simulink model "bike_model_pidTuning"  (R2018b)
settings: Solver=FixedStepAuto  StartTime=0.0  StopTime=sim_time  FixedStep=Ts_IMU  MaxStep=Ts  RelTol=1e-3
values from neighbouring files (symbols this model uses):
  a_compFilter = a_real    (= 0.4964)    [configuration_boxMovedCenter.m]    (also in configuration_lqrTuning.m = 0.325; configuration_pidTuning.m = 0.325; configuration_yixiao.m = 0.325)
  b_compFilter = b_real    (= 1.095)    [configuration_boxMovedCenter.m]    (also in configuration_lqrTuning.m; configuration_pidTuning.m; configuration_yixiao.m)
  b_real = 1.095    [configuration_boxMovedCenter.m]    (also in configuration_lqrTuning.m; configuration_pidTuning.m; configuration_yixiao.m)
  direct_control = 1    [configuration_boxMovedCenter.m]    (also in configuration_lqrTuning.m; configuration_pidTuning.m; configuration_yixiao.m)
  IMU_height_real = 0.45    [configuration_boxMovedCenter.m]    (also in configuration_lqrTuning.m; configuration_pidTuning.m; configuration_yixiao.m)
  initial_states = [deg2rad(5) deg2rad(-2) deg2rad(0)]    [configuration_boxMovedCenter.m]    (also in configuration_lqrTuning.m = [deg2rad(-2) deg2rad(0) deg2rad(0)]; configuration_pidTuning.m = [deg2rad(-2) deg2rad(0) deg2rad(0)]; configuration_yixiao.m = [deg2rad(-2) deg2rad(0) deg2rad(0)])
  input_velocity = 3    [configuration_boxMovedCenter.m]    (also in configuration_lqrTuning.m; configuration_pidTuning.m; configuration_yixiao.m)
  lambda_compFilter = deg2rad(70)    [configuration_boxMovedCenter.m]    (also in configuration_lqrTuning.m; configuration_pidTuning.m; configuration_yixiao.m)
  lambda_real = deg2rad(70)    [configuration_boxMovedCenter.m]    (also in configuration_lqrTuning.m; configuration_pidTuning.m; configuration_yixiao.m)
  look_ahead = 0    [configuration_boxMovedCenter.m]    (also in configuration_lqrTuning.m; configuration_pidTuning.m; configuration_yixiao.m)
  parameters_compFilter = [g h_compFilter b_compFilter a_compFilter lambda_compFilter c_compFilter]    [configuration_boxMovedCenter.m]    (also in configuration_lqrTuning.m; configuration_pidTuning.m; configuration_yixiao.m)
  parameters_f_b_real = [m_frame_real m_box_real h_frame_real h_box_real a_frame_real a_box_real c_frame_real c_box_real b_frame_real b_box_real l_frame_real l_box_real]    [configuration_boxMovedCenter.m]    (also in configuration_lqrTuning.m; configuration_pidTuning.m; configuration_yixiao.m = [m_frame_real m_box_real h_frame_real h_box_real a_frame_rea)
  parameters_real = [g h_real b_real a_real lambda_real c_real]    [configuration_boxMovedCenter.m]    (also in configuration_lqrTuning.m; configuration_pidTuning.m; configuration_yixiao.m)
  plant_model = 1    [configuration_boxMovedCenter.m]    (also in configuration_lqrTuning.m; configuration_pidTuning.m; configuration_yixiao.m)
  Ts = 0.04    [configuration_boxMovedCenter.m]    (also in configuration_lqrTuning.m; configuration_pidTuning.m; configuration_yixiao.m)
  Ts_IMU = 0.04    [configuration_boxMovedCenter.m]    (also in configuration_lqrTuning.m; configuration_pidTuning.m; configuration_yixiao.m)
undefined symbols (not defined in the file or in its folder): cumulative_dist_along_path, curvature, DiscIntNeverNeededParam, initial_x, initial_y, lqr_gains, path_x, path_y, sys_con, sys_dis, velocity_lqr
libraries: simulink x20, dspsigops x2
(part 3 of 3)

== matlab function bike_model_pidTuning/Physical Bike/Linear Bicycle Model with neglected fork angle (lambda=90deg, c=0) "THE SIMPLEST MODEL" ==
  data: states input; input input; xdot output; velocity input; disturbance input; parameters_real input; parameters_f_b_real input
function xdot = fcn(states,input,velocity,disturbance,parameters_real,parameters_f_b_real)

delta_d=input;
v=velocity;
d1=disturbance(1);
d2=disturbance(2);
d3=disturbance(3);

% 1=frame | 2=box
m1=parameters_f_b_real(1);
m2=parameters_f_b_real(2);
h1=parameters_f_b_real(3);
h2=parameters_f_b_real(4);
a1=parameters_f_b_real(5);
a2=parameters_f_b_real(6);
c1=parameters_f_b_real(7);
c2=parameters_f_b_real(8);
b1=parameters_f_b_real(9);
b2=parameters_f_b_real(10);
l1=parameters_f_b_real(11);
l2=parameters_f_b_real(12);

g=parameters_real(1);
%h=parameters_real(2);
b=parameters_real(3);
%a=parameters_real(4);
lambda=parameters_real(5);
c=parameters_real(6);

A=((m1/12)*((c1^2)+(b1^2)))+(m1*(h1^2))+((m2/12)*((c2^2)+(b2^2)))+(m2*(h2^2));
B=((m1/12)*((l1^2)+(b1^2)))-(m1*a1*h1)+((m2/12)*((c2^2)+(b2^2)))+(m2*a2*h2);
D=(((m1*h1)+(m2*h2))*(v^2))-(c*g*((m1*a1)-(m2*a2)));

phi=states(1);
delta=states(2);
phi_d=states(3);

xdot1=phi_d+d1;
xdot2=delta_d+d2;
xdot3=((((m1*h1)+(m2*h2))*g)/A)*phi+((D*sin(lambda))/(b*A))*delta+d3+((B*v*sin(lambda))/(b*A))*delta_d;

xdot=[xdot1 xdot2 xdot3];

== matlab function bike_model_pidTuning/Global Angles and Coordinates Calculator - Velocity/Measured Bike Angles to Global Angles/MATLAB Function ==
  data: v input; parameters_model input; delta input; psi_d output; beta output
function [psi_d, beta]  = fcn(v, parameters_model, delta)

b = parameters_model(3);
a = parameters_model(4);

beta = atan((a / (b)) * tan(delta));
psi_d = (v / a) * sin(beta);

== matlab function bike_model_pidTuning/Global Angles and Coordinates Calculator - Velocity/Measured Global Angles to Global Coordinates/MATLAB Function1 ==
  data: v input; psi input; Xdot output; beta input; Ydot output
function [Xdot, Ydot]  = fcn(v, psi, beta)

Xdot = v * cos(psi + beta);
Ydot = v * sin(psi + beta);

== matlab function bike_model_pidTuning/Physical Bike/Global Angles and Coordinates Calculator - Position/Measured Global Angles to Global Coordinates/MATLAB Function1 ==
  data: v input; psi input; Xdot output; beta input; Ydot output
function [Xdot, Ydot]  = fcn(v, psi, beta)

Xdot = v * cos(psi + beta);
Ydot = v * sin(psi + beta);
